simulink model "bingo_dec16_32k"  (R2018a)
settings: Solver=VariableStepDiscrete  StartTime=0.0  StopTime=10.0  RelTol=1e-3
undefined symbols (not defined in the file): pfb_coeff_gen_calc
libraries: xbsIndex_r4 x9772, casper_library_misc x15, xps_library x4, casper_library_delays x2
(part 3 of 49)

== system bingo_dec16_32k/bit_sel_xy_re ==
  shift : Inport
  sync : Inport  Port=2
  din64 : Inport  Port=3
  valid : Inport  Port=4
  Reinterpret : xbsIndex_r4/Reinterpret  force_arith_type=on  arith_type=Unsigned  force_bin_pt=on  bin_pt=0  block_type=reinterpret
  Terminator{1..32} (32 alike) : Terminator
  barrel_switcher : Subsystem  AncestorBlock=casper_library_reorder/barrel_switcher  mask(barrel_switcher){n_inputs=6, async=off}
      mask prompts: n_inputs "Number of Inputs: (2^?)"; async "Asynchronous operation"
      mask help:
      | Shifts input to right by amount specified on sel,
      | wrapping around into higher order bits.
      mask init:
      | barrel_switcher_init(gcb,...
      |     'n_inputs', n_inputs, ...
      |     'async', async);
      mask Help: eval('xlWeb(''http://casper.berkeley.edu/wiki/Barrel_switcher'')')
  bus_create : Subsystem  AncestorBlock=casper_library_flow_control/bus_create  mask(bus_create){inputNum=32}
      mask prompts: inputNum "Number of inputs:"
      mask init:
      | bus_create_init(gcb,...
      |     'inputNum', inputNum);
  bus_expand1 : Subsystem  AncestorBlock=casper_library_flow_control/bus_expand  mask(bus_expand){mode=divisions of equal size, outputNum=64, outputWidth=1, outputBinaryPt=0, outputArithmeticType=0, show_format=off, outputToWorkspace=off, variablePrefix=out, outputToModelAsWell=on}
      mask prompts: outputNum "Number of outputs:"; outputWidth "Output width:"; outputBinaryPt "Output binary point position:"; outputArithmeticType "Output arithmetic type (ufix=0, fix=1, bool=2):"; show_format "Print format string?"; outputToWorkspace "Output to workspace?"; variablePrefix "Variable name prefix:"; outputToModelAsWell "Output to model as well?"
      mask help:
      | Expands a 'bus' made using a bus_create or Xilinx
      | concat block.
      | The input will be divided into the specified number
      | of outputs with the specified arithmetic types.
      | Divisions are made from most significant bit.
      mask init: same as bingo_dec16_32k/bit_sel_xx/bus_expand1
      settings: AttributesFormatString=64 outputs
      mask TypeOptions mode: divisions of equal size | divisions of arbitrary size
      mask Callback mode: bus_expand_callback();
      mask Callback outputWidth: bus_expand_callback();
      mask Callback outputToWorkspace: bus_expand_callback();
  sync_out : Outport
  "dout32 " : Outport  Port=2
  valid_out : Outport  Port=3
  wires:
  bus_expand1/13(out52) -> barrel_switcher/15(In13)
  bus_expand1/42(out23) -> barrel_switcher/44(In42)
  bus_expand1/27(out38) -> barrel_switcher/29(In27)
  bus_expand1/26(out39) -> barrel_switcher/28(In26)
  bus_expand1/33(out32) -> barrel_switcher/35(In33)
  bus_expand1/44(out21) -> barrel_switcher/46(In44)
  bus_expand1/12(out53) -> barrel_switcher/14(In12)
  bus_expand1/35(out30) -> barrel_switcher/37(In35)
  bus_expand1/23(out42) -> barrel_switcher/25(In23)
  bus_expand1/45(out20) -> barrel_switcher/47(In45)
  bus_expand1/50(out15) -> barrel_switcher/52(In50)
  bus_expand1/56(out9) -> barrel_switcher/58(In56)
  sync/1 -> barrel_switcher/2(sync_in)
  bus_expand1/24(out41) -> barrel_switcher/26(In24)
  bus_expand1/58(out7) -> barrel_switcher/60(In58)
  bus_expand1/53(out12) -> barrel_switcher/55(In53)
  bus_expand1/29(out36) -> barrel_switcher/31(In29)
  bus_expand1/43(out22) -> barrel_switcher/45(In43)
  bus_expand1/3(out62) -> barrel_switcher/5(In3)
  bus_expand1/61(out4) -> barrel_switcher/63(In61)
  bus_expand1/1(msb_out64) -> barrel_switcher/3(In1)
  bus_expand1/28(out37) -> barrel_switcher/30(In28)
  Reinterpret/1 -> bus_expand1/1(bus_in)
  bus_expand1/8(out57) -> barrel_switcher/10(In8)
  bus_expand1/20(out45) -> barrel_switcher/22(In20)
  bus_expand1/59(out6) -> barrel_switcher/61(In59)
  bus_expand1/30(out35) -> barrel_switcher/32(In30)
  bus_expand1/19(out46) -> barrel_switcher/21(In19)
  bus_expand1/9(out56) -> barrel_switcher/11(In9)
  bus_expand1/11(out54) -> barrel_switcher/13(In11)
  bus_expand1/18(out47) -> barrel_switcher/20(In18)
  bus_expand1/25(out40) -> barrel_switcher/27(In25)
  bus_expand1/32(out33) -> barrel_switcher/34(In32)
  bus_expand1/62(out3) -> barrel_switcher/64(In62)
  bus_expand1/37(out28) -> barrel_switcher/39(In37)
  bus_expand1/36(out29) -> barrel_switcher/38(In36)
  bus_expand1/41(out24) -> barrel_switcher/43(In41)
  bus_expand1/22(out43) -> barrel_switcher/24(In22)
  bus_expand1/48(out17) -> barrel_switcher/50(In48)
  bus_expand1/7(out58) -> barrel_switcher/9(In7)
  bus_expand1/63(out2) -> barrel_switcher/65(In63)
  bus_expand1/15(out50) -> barrel_switcher/17(In15)
  bus_expand1/49(out16) -> barrel_switcher/51(In49)
  shift/1 -> barrel_switcher/1(sel)
  bus_expand1/21(out44) -> barrel_switcher/23(In21)
  bus_expand1/46(out19) -> barrel_switcher/48(In46)
  bus_expand1/52(out13) -> barrel_switcher/54(In52)
  bus_expand1/54(out11) -> barrel_switcher/56(In54)
  bus_expand1/4(out61) -> barrel_switcher/6(In4)
  bus_expand1/31(out34) -> barrel_switcher/33(In31)
  bus_expand1/40(out25) -> barrel_switcher/42(In40)
  bus_expand1/39(out26) -> barrel_switcher/41(In39)
  bus_expand1/51(out14) -> barrel_switcher/53(In51)
  bus_expand1/64(lsb_out1) -> barrel_switcher/66(In64)
  bus_expand1/38(out27) -> barrel_switcher/40(In38)
  din64/1 -> Reinterpret/1
  bus_expand1/5(out60) -> barrel_switcher/7(In5)
  bus_expand1/17(out48) -> barrel_switcher/19(In17)
  bus_expand1/16(out49) -> barrel_switcher/18(In16)
  bus_expand1/10(out55) -> barrel_switcher/12(In10)
  bus_expand1/14(out51) -> barrel_switcher/16(In14)
  bus_expand1/2(out63) -> barrel_switcher/4(In2)
  bus_expand1/60(out5) -> barrel_switcher/62(In60)
  bus_expand1/55(out10) -> barrel_switcher/57(In55)
  bus_expand1/6(out59) -> barrel_switcher/8(In6)
  bus_expand1/47(out18) -> barrel_switcher/49(In47)
  bus_expand1/57(out8) -> barrel_switcher/59(In57)
  bus_expand1/34(out31) -> barrel_switcher/36(In34)
  bus_create/1(bus_out) -> "dout32 "/1
  barrel_switcher/1(sync_out) -> sync_out/1
  barrel_switcher/66(valid_out) -> valid_out/1
  valid/1 -> barrel_switcher/67(valid_in)
  barrel_switcher/35(Out34) -> Terminator1/1
  barrel_switcher/40(Out39) -> Terminator7/1
  barrel_switcher/45(Out44) -> Terminator11/1
  barrel_switcher/56(Out55) -> Terminator30/1
  barrel_switcher/42(Out41) -> Terminator9/1
  barrel_switcher/64(Out63) -> Terminator24/1
  barrel_switcher/47(Out46) -> Terminator13/1
  barrel_switcher/58(Out57) -> Terminator32/1
  barrel_switcher/61(Out60) -> Terminator19/1
  barrel_switcher/37(Out36) -> Terminator2/1
  barrel_switcher/36(Out35) -> Terminator3/1
  barrel_switcher/53(Out52) -> Terminator25/1
  barrel_switcher/51(Out50) -> Terminator17/1
  barrel_switcher/43(Out42) -> Terminator8/1
  barrel_switcher/62(Out61) -> Terminator22/1
  barrel_switcher/50(Out49) -> Terminator18/1
  barrel_switcher/57(Out56) -> Terminator29/1
  barrel_switcher/49(Out48) -> Terminator15/1
  barrel_switcher/55(Out54) -> Terminator27/1
  barrel_switcher/52(Out51) -> Terminator26/1
  barrel_switcher/60(Out59) -> Terminator20/1
  barrel_switcher/46(Out45) -> Terminator14/1
  barrel_switcher/63(Out62) -> Terminator21/1
  barrel_switcher/65(Out64) -> Terminator23/1
  barrel_switcher/34(Out33) -> Terminator10/1
  barrel_switcher/54(Out53) -> Terminator28/1
  barrel_switcher/41(Out40) -> Terminator6/1
  barrel_switcher/59(Out58) -> Terminator31/1
  barrel_switcher/38(Out37) -> Terminator5/1
  barrel_switcher/44(Out43) -> Terminator12/1
  barrel_switcher/39(Out38) -> Terminator4/1
  barrel_switcher/48(Out47) -> Terminator16/1
  barrel_switcher/2(Out1) -> bus_create/1(in1)
  barrel_switcher/3(Out2) -> bus_create/2(in2)
  barrel_switcher/4(Out3) -> bus_create/3(in3)
  barrel_switcher/5(Out4) -> bus_create/4(in4)
  barrel_switcher/6(Out5) -> bus_create/5(in5)
  barrel_switcher/7(Out6) -> bus_create/6(in6)
  barrel_switcher/8(Out7) -> bus_create/7(in7)
  barrel_switcher/9(Out8) -> bus_create/8(in8)
  barrel_switcher/10(Out9) -> bus_create/9(in9)
  barrel_switcher/11(Out10) -> bus_create/10(in10)
  barrel_switcher/12(Out11) -> bus_create/11(in11)
  barrel_switcher/13(Out12) -> bus_create/12(in12)
  barrel_switcher/14(Out13) -> bus_create/13(in13)
  barrel_switcher/15(Out14) -> bus_create/14(in14)
  barrel_switcher/16(Out15) -> bus_create/15(in15)
  barrel_switcher/17(Out16) -> bus_create/16(in16)
  barrel_switcher/18(Out17) -> bus_create/17(in17)
  barrel_switcher/19(Out18) -> bus_create/18(in18)
  barrel_switcher/20(Out19) -> bus_create/19(in19)
  barrel_switcher/21(Out20) -> bus_create/20(in20)
  barrel_switcher/22(Out21) -> bus_create/21(in21)
  barrel_switcher/23(Out22) -> bus_create/22(in22)
  barrel_switcher/24(Out23) -> bus_create/23(in23)
  barrel_switcher/25(Out24) -> bus_create/24(in24)
  barrel_switcher/26(Out25) -> bus_create/25(in25)
  barrel_switcher/27(Out26) -> bus_create/26(in26)
  barrel_switcher/28(Out27) -> bus_create/27(in27)
  barrel_switcher/29(Out28) -> bus_create/28(in28)
  barrel_switcher/30(Out29) -> bus_create/29(in29)
  barrel_switcher/31(Out30) -> bus_create/30(in30)
  barrel_switcher/32(Out31) -> bus_create/31(in31)
  barrel_switcher/33(Out32) -> bus_create/32(in32)

== system bingo_dec16_32k/bit_sel_yy ==
  shift : Inport
  sync : Inport  Port=2
  din64 : Inport  Port=3
  valid : Inport  Port=4
  Reinterpret : xbsIndex_r4/Reinterpret  force_arith_type=on  arith_type=Unsigned  force_bin_pt=on  bin_pt=0  block_type=reinterpret
  Terminator{1..32} (32 alike) : Terminator
  barrel_switcher : Subsystem  AncestorBlock=casper_library_reorder/barrel_switcher  mask(barrel_switcher){n_inputs=6, async=off}
      mask prompts: n_inputs "Number of Inputs: (2^?)"; async "Asynchronous operation"
      mask help:
      | Shifts input to right by amount specified on sel,
      | wrapping around into higher order bits.
      mask init:
      | barrel_switcher_init(gcb,...
      |     'n_inputs', n_inputs, ...
      |     'async', async);
      mask Help: eval('xlWeb(''http://casper.berkeley.edu/wiki/Barrel_switcher'')')
  bus_create : Subsystem  AncestorBlock=casper_library_flow_control/bus_create  mask(bus_create){inputNum=32}
      mask prompts: inputNum "Number of inputs:"
      mask init:
      | bus_create_init(gcb,...
      |     'inputNum', inputNum);
  bus_expand1 : Subsystem  AncestorBlock=casper_library_flow_control/bus_expand  mask(bus_expand){mode=divisions of equal size, outputNum=64, outputWidth=1, outputBinaryPt=0, outputArithmeticType=0, show_format=off, outputToWorkspace=off, variablePrefix=out, outputToModelAsWell=on}
      mask prompts: outputNum "Number of outputs:"; outputWidth "Output width:"; outputBinaryPt "Output binary point position:"; outputArithmeticType "Output arithmetic type (ufix=0, fix=1, bool=2):"; show_format "Print format string?"; outputToWorkspace "Output to workspace?"; variablePrefix "Variable name prefix:"; outputToModelAsWell "Output to model as well?"
      mask help:
      | Expands a 'bus' made using a bus_create or Xilinx
      | concat block.
      | The input will be divided into the specified number
      | of outputs with the specified arithmetic types.
      | Divisions are made from most significant bit.
      mask init: same as bingo_dec16_32k/bit_sel_xx/bus_expand1
      settings: AttributesFormatString=64 outputs
      mask TypeOptions mode: divisions of equal size | divisions of arbitrary size
      mask Callback mode: bus_expand_callback();
      mask Callback outputWidth: bus_expand_callback();
      mask Callback outputToWorkspace: bus_expand_callback();
  sync_out : Outport
  "dout32 " : Outport  Port=2
  valid_out : Outport  Port=3
  wires:
  bus_expand1/13(out52) -> barrel_switcher/15(In13)
  bus_expand1/42(out23) -> barrel_switcher/44(In42)
  bus_expand1/27(out38) -> barrel_switcher/29(In27)
  bus_expand1/26(out39) -> barrel_switcher/28(In26)
  bus_expand1/33(out32) -> barrel_switcher/35(In33)
  bus_expand1/44(out21) -> barrel_switcher/46(In44)
  bus_expand1/12(out53) -> barrel_switcher/14(In12)
  bus_expand1/35(out30) -> barrel_switcher/37(In35)
  bus_expand1/23(out42) -> barrel_switcher/25(In23)
  bus_expand1/45(out20) -> barrel_switcher/47(In45)
  bus_expand1/50(out15) -> barrel_switcher/52(In50)
  bus_expand1/56(out9) -> barrel_switcher/58(In56)
  sync/1 -> barrel_switcher/2(sync_in)
  bus_expand1/24(out41) -> barrel_switcher/26(In24)
  bus_expand1/58(out7) -> barrel_switcher/60(In58)
  bus_expand1/53(out12) -> barrel_switcher/55(In53)
  bus_expand1/29(out36) -> barrel_switcher/31(In29)
  bus_expand1/43(out22) -> barrel_switcher/45(In43)
  bus_expand1/3(out62) -> barrel_switcher/5(In3)
  bus_expand1/61(out4) -> barrel_switcher/63(In61)
  bus_expand1/1(msb_out64) -> barrel_switcher/3(In1)
  bus_expand1/28(out37) -> barrel_switcher/30(In28)
  Reinterpret/1 -> bus_expand1/1(bus_in)
  bus_expand1/8(out57) -> barrel_switcher/10(In8)
  bus_expand1/20(out45) -> barrel_switcher/22(In20)
  bus_expand1/59(out6) -> barrel_switcher/61(In59)
  bus_expand1/30(out35) -> barrel_switcher/32(In30)
  bus_expand1/19(out46) -> barrel_switcher/21(In19)
  bus_expand1/9(out56) -> barrel_switcher/11(In9)
  bus_expand1/11(out54) -> barrel_switcher/13(In11)
  bus_expand1/18(out47) -> barrel_switcher/20(In18)
  bus_expand1/25(out40) -> barrel_switcher/27(In25)
  bus_expand1/32(out33) -> barrel_switcher/34(In32)
  bus_expand1/62(out3) -> barrel_switcher/64(In62)
  bus_expand1/37(out28) -> barrel_switcher/39(In37)
  bus_expand1/36(out29) -> barrel_switcher/38(In36)
  bus_expand1/41(out24) -> barrel_switcher/43(In41)
  bus_expand1/22(out43) -> barrel_switcher/24(In22)
  bus_expand1/48(out17) -> barrel_switcher/50(In48)
  bus_expand1/7(out58) -> barrel_switcher/9(In7)
  bus_expand1/63(out2) -> barrel_switcher/65(In63)
  bus_expand1/15(out50) -> barrel_switcher/17(In15)
  bus_expand1/49(out16) -> barrel_switcher/51(In49)
  shift/1 -> barrel_switcher/1(sel)
  bus_expand1/21(out44) -> barrel_switcher/23(In21)
  bus_expand1/46(out19) -> barrel_switcher/48(In46)
  bus_expand1/52(out13) -> barrel_switcher/54(In52)
  bus_expand1/54(out11) -> barrel_switcher/56(In54)
  bus_expand1/4(out61) -> barrel_switcher/6(In4)
  bus_expand1/31(out34) -> barrel_switcher/33(In31)
  bus_expand1/40(out25) -> barrel_switcher/42(In40)
  bus_expand1/39(out26) -> barrel_switcher/41(In39)
  bus_expand1/51(out14) -> barrel_switcher/53(In51)
  bus_expand1/64(lsb_out1) -> barrel_switcher/66(In64)
  bus_expand1/38(out27) -> barrel_switcher/40(In38)
  din64/1 -> Reinterpret/1
  bus_expand1/5(out60) -> barrel_switcher/7(In5)
  bus_expand1/17(out48) -> barrel_switcher/19(In17)
  bus_expand1/16(out49) -> barrel_switcher/18(In16)
  bus_expand1/10(out55) -> barrel_switcher/12(In10)
  bus_expand1/14(out51) -> barrel_switcher/16(In14)
  bus_expand1/2(out63) -> barrel_switcher/4(In2)
  bus_expand1/60(out5) -> barrel_switcher/62(In60)
  bus_expand1/55(out10) -> barrel_switcher/57(In55)
  bus_expand1/6(out59) -> barrel_switcher/8(In6)
  bus_expand1/47(out18) -> barrel_switcher/49(In47)
  bus_expand1/57(out8) -> barrel_switcher/59(In57)
  bus_expand1/34(out31) -> barrel_switcher/36(In34)
  bus_create/1(bus_out) -> "dout32 "/1
  barrel_switcher/1(sync_out) -> sync_out/1
  barrel_switcher/66(valid_out) -> valid_out/1
  valid/1 -> barrel_switcher/67(valid_in)
  barrel_switcher/35(Out34) -> Terminator1/1
  barrel_switcher/40(Out39) -> Terminator7/1
  barrel_switcher/45(Out44) -> Terminator11/1
  barrel_switcher/56(Out55) -> Terminator30/1
  barrel_switcher/42(Out41) -> Terminator9/1
  barrel_switcher/64(Out63) -> Terminator24/1
  barrel_switcher/47(Out46) -> Terminator13/1
  barrel_switcher/58(Out57) -> Terminator32/1
  barrel_switcher/61(Out60) -> Terminator19/1
  barrel_switcher/37(Out36) -> Terminator2/1
  barrel_switcher/36(Out35) -> Terminator3/1
  barrel_switcher/53(Out52) -> Terminator25/1
  barrel_switcher/51(Out50) -> Terminator17/1
  barrel_switcher/43(Out42) -> Terminator8/1
  barrel_switcher/62(Out61) -> Terminator22/1
  barrel_switcher/50(Out49) -> Terminator18/1
  barrel_switcher/57(Out56) -> Terminator29/1
  barrel_switcher/49(Out48) -> Terminator15/1
  barrel_switcher/55(Out54) -> Terminator27/1
  barrel_switcher/52(Out51) -> Terminator26/1
  barrel_switcher/60(Out59) -> Terminator20/1
  barrel_switcher/46(Out45) -> Terminator14/1
  barrel_switcher/63(Out62) -> Terminator21/1
  barrel_switcher/65(Out64) -> Terminator23/1
  barrel_switcher/34(Out33) -> Terminator10/1
  barrel_switcher/54(Out53) -> Terminator28/1
  barrel_switcher/41(Out40) -> Terminator6/1
  barrel_switcher/59(Out58) -> Terminator31/1
  barrel_switcher/38(Out37) -> Terminator5/1
  barrel_switcher/44(Out43) -> Terminator12/1
  barrel_switcher/39(Out38) -> Terminator4/1
  barrel_switcher/48(Out47) -> Terminator16/1
  barrel_switcher/2(Out1) -> bus_create/1(in1)
  barrel_switcher/3(Out2) -> bus_create/2(in2)
  barrel_switcher/4(Out3) -> bus_create/3(in3)
  barrel_switcher/5(Out4) -> bus_create/4(in4)
  barrel_switcher/6(Out5) -> bus_create/5(in5)
  barrel_switcher/7(Out6) -> bus_create/6(in6)
  barrel_switcher/8(Out7) -> bus_create/7(in7)
  barrel_switcher/9(Out8) -> bus_create/8(in8)
  barrel_switcher/10(Out9) -> bus_create/9(in9)
  barrel_switcher/11(Out10) -> bus_create/10(in10)
  barrel_switcher/12(Out11) -> bus_create/11(in11)
  barrel_switcher/13(Out12) -> bus_create/12(in12)
  barrel_switcher/14(Out13) -> bus_create/13(in13)
  barrel_switcher/15(Out14) -> bus_create/14(in14)
  barrel_switcher/16(Out15) -> bus_create/15(in15)
  barrel_switcher/17(Out16) -> bus_create/16(in16)
  barrel_switcher/18(Out17) -> bus_create/17(in17)
  barrel_switcher/19(Out18) -> bus_create/18(in18)
  barrel_switcher/20(Out19) -> bus_create/19(in19)
  barrel_switcher/21(Out20) -> bus_create/20(in20)
  barrel_switcher/22(Out21) -> bus_create/21(in21)
  barrel_switcher/23(Out22) -> bus_create/22(in22)
  barrel_switcher/24(Out23) -> bus_create/23(in23)
  barrel_switcher/25(Out24) -> bus_create/24(in24)
  barrel_switcher/26(Out25) -> bus_create/25(in25)
  barrel_switcher/27(Out26) -> bus_create/26(in26)
  barrel_switcher/28(Out27) -> bus_create/27(in27)
  barrel_switcher/29(Out28) -> bus_create/28(in28)
  barrel_switcher/30(Out29) -> bus_create/29(in29)
  barrel_switcher/31(Out30) -> bus_create/30(in30)
  barrel_switcher/32(Out31) -> bus_create/31(in31)
  barrel_switcher/33(Out32) -> bus_create/32(in32)

== system bingo_dec16_32k/bus_create ==
  in1 : Inport
  in2 : Inport  Port=2
  in3 : Inport  Port=3
  in4 : Inport  Port=4
  concatenate : xbsIndex_r4/Concat  num_inputs=4  dbl_ovrd=off  block_type=concat
  reinterpret{1..4} (4 alike) : xbsIndex_r4/Reinterpret  force_arith_type=on  arith_type=Unsigned  force_bin_pt=on  bin_pt=0  block_type=reinterpret
      reinterpret1 settings: infoedit="Changes signal type without altering the binary representation.   You can changed the signal between signed and unsigned, and relocate the binary point.<br><br>Hardware notes: In hardware this block costs nothing.<br><br>Example:  Suppose the input is 6 bits wide, signed, with 2 fractional bits, and the output is forced to unsigned with 0 fractional bits.  Then an input of -2.0 (1110.00 in binary 2's complement) becomes an output of 56 (111000 in binary)."
      reinterpret2 settings: infoedit="Changes signal type without altering the binary representation.   You can changed the signal between signed and unsigned, and relocate the binary point.<br><br>Hardware notes: In hardware this block costs nothing.<br><br>Example:  Suppose the input is 6 bits wide, signed, with 2 fractional bits, and the output is forced to unsigned with 0 fractional bits.  Then an input of -2.0 (1110.00 in binary 2's complement) becomes an output of 56 (111000 in binary)."
  bus_out : Outport
  wires:
  concatenate/1 -> bus_out/1
  in1/1 -> reinterpret1/1
  reinterpret1/1 -> concatenate/1
  in2/1 -> reinterpret2/1
  reinterpret2/1 -> concatenate/2
  in3/1 -> reinterpret3/1
  reinterpret3/1 -> concatenate/3
  in4/1 -> reinterpret4/1
  reinterpret4/1 -> concatenate/4

== system bingo_dec16_32k/calc_adc_sum_sq1 ==
  In1 : Inport
  In2 : Inport  Port=2
  "valid " : Inport  Port=3
  Accumulator : xbsIndex_r4/Accumulator  operation=Add  n_bits=47  overflow=Wrap  scale=1  rst=on  hasbypass=on  infoeditControl=reset for floating point data type must be asserted for a minimum of 2 cycles  en=on  latency=0  msb_inp=100  msb=100  lsb=-100  use_behavioral_HDL=off  implementation=DSP48  dbl_ovrd=off  block_type=accum
      settings: xl_area=[0, 0, 0, 0, 0, 0, 0]  block_version=10.1.3
  AddSub9 : xbsIndex_r4/AddSub  mode=Addition  use_carryin=off  use_carryout=off  en=off  latency=1  precision=Full  arith_type=Unsigned  n_bits=16  bin_pt=14  quantization=Truncate  overflow=Wrap  use_behavioral_HDL=off  hw_selection=Fabric  pipelined=off  dbl_ovrd=off  block_type=addsub
  Convert1 : xbsIndex_r4/Convert  gui_display_data_type=Fixed-point  arith_type=Unsigned  n_bits=32  bin_pt=15  float_type=Single  exp_bits=8  fraction_bits=24  quantization=Truncate  overflow=Wrap  en=off  latency=0  pipeline=off  dbl_ovrd=off  block_type=convert
      settings: block_version=11.4
  Counter1 : xbsIndex_r4/Counter  cnt_type=Free Running  cnt_to=Inf  operation=Up  start_count=0  cnt_by_val=1  arith_type=Unsigned  n_bits=16  bin_pt=0  load_pin=off  rst=off  en=on  explicit_period=on  period=1  use_behavioral_HDL=off  implementation=DSP48  use_rpm=on  dbl_ovrd=off  block_type=counter
      settings: xl_area=[0, 0, 0, 0, 0, 0, 0]
  Delay : xbsIndex_r4/Delay  rst=off  infoeditControl=Selection of Reset will increase slice count due to use of real FFs and instead of SRLs  en=off  latency=3  reg_retiming=off  dbl_ovrd=off  block_type=delay
  Delay1 : xbsIndex_r4/Delay  rst=off  infoeditControl=Selection of Reset will increase slice count due to use of real FFs and instead of SRLs  en=off  latency=2  reg_retiming=on  dbl_ovrd=off  block_type=delay
      settings: block_version=11.4
  Logical : xbsIndex_r4/Logical  logical_function=AND  inputs=2  en=off  latency=0  precision=Full  arith_type=Unsigned  n_bits=16  bin_pt=0  align_bp=on  dbl_ovrd=off  block_type=logical
  Mult : xbsIndex_r4/Mult  precision=Full  arith_type="Signed  (2's comp)"  n_bits=8  bin_pt=2  quantization=Truncate  overflow=Wrap  en=off  latency=2  use_behavioral_HDL=on  opt=Speed  use_embedded=on  optimum_pipeline=off  pipeline=on  dbl_ovrd=off  use_rpm=on  placement_style=Rectangular shape  block_type=mult
      settings: xl_area=[0, 0, 0, 0, 0, 0, 0]  block_version=10.1.3
  Mult8 : xbsIndex_r4/Mult  precision=Full  arith_type="Signed  (2's comp)"  n_bits=8  bin_pt=2  quantization=Truncate  overflow=Wrap  en=off  latency=2  use_behavioral_HDL=on  opt=Speed  use_embedded=on  optimum_pipeline=off  pipeline=on  dbl_ovrd=off  use_rpm=on  placement_style=Rectangular shape  block_type=mult
      settings: xl_area=[0, 0, 0, 0, 0, 0, 0]  block_version=10.1.3
  Register : xbsIndex_r4/Register  init=0  rst=off  en=on  dbl_ovrd=off  block_type=register
      settings: xl_area=[0, 0, 0, 0, 0, 0, 0]
  Slice : xbsIndex_r4/Slice  nbits=1  boolean_output=off  mode=Upper Bit Location + Width  bit1=0  base1=MSB of Input  bit0=0  base0=LSB of Input  dbl_ovrd=off  block_type=slice
      settings: infoedit="Extracts a given range of bits from each input sample and presents it at the output.  The output type is ordinarily unsigned with binary point at zero, but can be Boolean when the slice is one bit wide.<P><P>Hardware notes: In hardware this block costs nothing."  block_version=10.1.3
  negedge : Subsystem
  sum_sq : Outport
  wires:
  Accumulator/1 -> Register/1
  Register/1 -> Convert1/1
  In2/1 -> Mult/1, Mult/2
  Counter1/1 -> Slice/1
  Slice/1 -> negedge/1(In)
  negedge/1(Out1) -> Delay1/1
  Convert1/1 -> sum_sq/1
  AddSub9/1 -> Accumulator/1
  Delay1/1 -> Logical/2
  In1/1 -> Mult8/1, Mult8/2
  Mult8/1 -> AddSub9/1
  Mult/1 -> AddSub9/2
  "valid "/1 -> Counter1/1, Delay/1
  Delay/1 -> Logical/1, Accumulator/3
  Logical/1 -> Register/2, Accumulator/2

== system bingo_dec16_32k/calc_adc_sum_sq2 ==
  In1 : Inport
  In2 : Inport  Port=2
  "valid " : Inport  Port=3
  Accumulator : xbsIndex_r4/Accumulator  operation=Add  n_bits=47  overflow=Wrap  scale=1  rst=on  hasbypass=on  infoeditControl=reset for floating point data type must be asserted for a minimum of 2 cycles  en=on  latency=0  msb_inp=100  msb=100  lsb=-100  use_behavioral_HDL=off  implementation=DSP48  dbl_ovrd=off  block_type=accum
      settings: xl_area=[0, 0, 0, 0, 0, 0, 0]  block_version=10.1.3
  AddSub9 : xbsIndex_r4/AddSub  mode=Addition  use_carryin=off  use_carryout=off  en=off  latency=1  precision=Full  arith_type=Unsigned  n_bits=16  bin_pt=14  quantization=Truncate  overflow=Wrap  use_behavioral_HDL=off  hw_selection=Fabric  pipelined=off  dbl_ovrd=off  block_type=addsub
  Convert1 : xbsIndex_r4/Convert  gui_display_data_type=Fixed-point  arith_type=Unsigned  n_bits=32  bin_pt=15  float_type=Single  exp_bits=8  fraction_bits=24  quantization=Truncate  overflow=Wrap  en=off  latency=0  pipeline=off  dbl_ovrd=off  block_type=convert
      settings: block_version=11.4
  Counter1 : xbsIndex_r4/Counter  cnt_type=Free Running  cnt_to=Inf  operation=Up  start_count=0  cnt_by_val=1  arith_type=Unsigned  n_bits=16  bin_pt=0  load_pin=off  rst=off  en=on  explicit_period=on  period=1  use_behavioral_HDL=off  implementation=DSP48  use_rpm=on  dbl_ovrd=off  block_type=counter
      settings: xl_area=[0, 0, 0, 0, 0, 0, 0]
  Delay : xbsIndex_r4/Delay  rst=off  infoeditControl=Selection of Reset will increase slice count due to use of real FFs and instead of SRLs  en=off  latency=3  reg_retiming=off  dbl_ovrd=off  block_type=delay
  Delay1 : xbsIndex_r4/Delay  rst=off  infoeditControl=Selection of Reset will increase slice count due to use of real FFs and instead of SRLs  en=off  latency=2  reg_retiming=on  dbl_ovrd=off  block_type=delay
      settings: block_version=11.4
  Logical : xbsIndex_r4/Logical  logical_function=AND  inputs=2  en=off  latency=0  precision=Full  arith_type=Unsigned  n_bits=16  bin_pt=0  align_bp=on  dbl_ovrd=off  block_type=logical
  Mult : xbsIndex_r4/Mult  precision=Full  arith_type="Signed  (2's comp)"  n_bits=8  bin_pt=2  quantization=Truncate  overflow=Wrap  en=off  latency=2  use_behavioral_HDL=on  opt=Speed  use_embedded=on  optimum_pipeline=off  pipeline=on  dbl_ovrd=off  use_rpm=on  placement_style=Rectangular shape  block_type=mult
      settings: xl_area=[0, 0, 0, 0, 0, 0, 0]  block_version=10.1.3
  Mult8 : xbsIndex_r4/Mult  precision=Full  arith_type="Signed  (2's comp)"  n_bits=8  bin_pt=2  quantization=Truncate  overflow=Wrap  en=off  latency=2  use_behavioral_HDL=on  opt=Speed  use_embedded=on  optimum_pipeline=off  pipeline=on  dbl_ovrd=off  use_rpm=on  placement_style=Rectangular shape  block_type=mult
      settings: xl_area=[0, 0, 0, 0, 0, 0, 0]  block_version=10.1.3
  Register : xbsIndex_r4/Register  init=0  rst=off  en=on  dbl_ovrd=off  block_type=register
      settings: xl_area=[0, 0, 0, 0, 0, 0, 0]
  Slice : xbsIndex_r4/Slice  nbits=1  boolean_output=off  mode=Upper Bit Location + Width  bit1=0  base1=MSB of Input  bit0=0  base0=LSB of Input  dbl_ovrd=off  block_type=slice
      settings: infoedit="Extracts a given range of bits from each input sample and presents it at the output.  The output type is ordinarily unsigned with binary point at zero, but can be Boolean when the slice is one bit wide.<P><P>Hardware notes: In hardware this block costs nothing."  block_version=10.1.3
  negedge : Subsystem
  sum_sq : Outport
  wires:
  Accumulator/1 -> Register/1
  Register/1 -> Convert1/1
  In2/1 -> Mult/1, Mult/2
  Counter1/1 -> Slice/1
  Slice/1 -> negedge/1(In)
  negedge/1(Out1) -> Delay1/1
  Convert1/1 -> sum_sq/1
  AddSub9/1 -> Accumulator/1
  Delay1/1 -> Logical/2
  In1/1 -> Mult8/1, Mult8/2
  Mult8/1 -> AddSub9/1
  Mult/1 -> AddSub9/2
  "valid "/1 -> Counter1/1, Delay/1
  Delay/1 -> Logical/1, Accumulator/3
  Logical/1 -> Register/2, Accumulator/2

== system bingo_dec16_32k/center_freq ==
  sim_1 : Inport
  bingo_dec16_32k_center_freq_user_data_out : xbsIndex_r4/Gateway In  gui_display_data_type=Fixed-point  arith_type=Unsigned  n_bits=32  bin_pt=0  preci_type=Single  exp_width=8  frac_width=24  rows=1  columns=1  quantization="Round  (unbiased: +/- Inf)"  overflow=Saturate  period=1  UseAsADC=off  ADCChannel='1'  interface=None  automatic_assignment=on  address_offset=hex2dec('00')  intf_name=''  intf_description=''  default_value=0  timing_constraint=None  locs_specified=off  LOCs={}  io_standard={}  inherit_from_input=off  hdl_port=on  dbl_ovrd=off  block_type=gatewayin
  convert1_1 : DataTypeConversion  OutDataTypeStr=fixdt('ufix32_En0')  LockScale=on
  convert2_1 : DataTypeConversion  OutDataTypeStr=fixdt('ufix32_En0')  ConvertRealWorld=Stored Integer (SI)  LockScale=on
  gain_1 : Gain
  io_delay : xbsIndex_r4/Delay  rst=off  infoeditControl=Selection of Reset will increase slice count due to use of real FFs and instead of SRLs  en=off  latency=0  reg_retiming=on  dbl_ovrd=off  block_type=delay
  reint1 : xbsIndex_r4/Reinterpret  force_arith_type=on  arith_type=Unsigned  force_bin_pt=on  bin_pt=0  block_type=reinterpret
  slice_reg : xbsIndex_r4/Slice  nbits=32  boolean_output=off  mode=Lower Bit Location + Width  bit1=0  base1=MSB of Input  bit0=0  base0=LSB of Input  dbl_ovrd=off  block_type=slice
  in_reg : Outport
  wires:
  bingo_dec16_32k_center_freq_user_data_out/1 -> io_delay/1
  sim_1/1 -> convert1_1/1
  convert1_1/1 -> convert2_1/1
  convert2_1/1 -> gain_1/1
  gain_1/1 -> bingo_dec16_32k_center_freq_user_data_out/1
  io_delay/1 -> slice_reg/1
  slice_reg/1 -> reint1/1
  reint1/1 -> in_reg/1

== system bingo_dec16_32k/clr_bc ==
  sim_1 : Inport
  bingo_dec16_32k_clr_bc_user_data_out : xbsIndex_r4/Gateway In  gui_display_data_type=Fixed-point  arith_type=Unsigned  n_bits=32  bin_pt=0  preci_type=Single  exp_width=8  frac_width=24  rows=1  columns=1  quantization="Round  (unbiased: +/- Inf)"  overflow=Saturate  period=1  UseAsADC=off  ADCChannel='1'  interface=None  automatic_assignment=on  address_offset=hex2dec('00')  intf_name=''  intf_description=''  default_value=0  timing_constraint=None  locs_specified=off  LOCs={}  io_standard={}  inherit_from_input=off  hdl_port=on  dbl_ovrd=off  block_type=gatewayin
  convert1_1 : DataTypeConversion  OutDataTypeStr=fixdt('ufix32_En0')  LockScale=on
  convert2_1 : DataTypeConversion  OutDataTypeStr=fixdt('ufix32_En0')  ConvertRealWorld=Stored Integer (SI)  LockScale=on
  gain_1 : Gain
  io_delay : xbsIndex_r4/Delay  rst=off  infoeditControl=Selection of Reset will increase slice count due to use of real FFs and instead of SRLs  en=off  latency=0  reg_retiming=on  dbl_ovrd=off  block_type=delay
  reint1 : xbsIndex_r4/Reinterpret  force_arith_type=on  arith_type=Unsigned  force_bin_pt=on  bin_pt=0  block_type=reinterpret
  slice_reg : xbsIndex_r4/Slice  nbits=32  boolean_output=off  mode=Lower Bit Location + Width  bit1=0  base1=MSB of Input  bit0=0  base0=LSB of Input  dbl_ovrd=off  block_type=slice
  in_reg : Outport
  wires:
  bingo_dec16_32k_clr_bc_user_data_out/1 -> io_delay/1
  sim_1/1 -> convert1_1/1
  convert1_1/1 -> convert2_1/1
  convert2_1/1 -> gain_1/1
  gain_1/1 -> bingo_dec16_32k_clr_bc_user_data_out/1
  io_delay/1 -> slice_reg/1
  slice_reg/1 -> reint1/1
  reint1/1 -> in_reg/1

== system bingo_dec16_32k/cnt_rst ==
  sim_1 : Inport
  bingo_dec16_32k_cnt_rst_user_data_out : xbsIndex_r4/Gateway In  gui_display_data_type=Fixed-point  arith_type=Unsigned  n_bits=32  bin_pt=0  preci_type=Single  exp_width=8  frac_width=24  rows=1  columns=1  quantization="Round  (unbiased: +/- Inf)"  overflow=Saturate  period=1  UseAsADC=off  ADCChannel='1'  interface=None  automatic_assignment=on  address_offset=hex2dec('00')  intf_name=''  intf_description=''  default_value=0  timing_constraint=None  locs_specified=off  LOCs={}  io_standard={}  inherit_from_input=off  hdl_port=on  dbl_ovrd=off  block_type=gatewayin
  convert1_1 : DataTypeConversion  OutDataTypeStr=fixdt('ufix32_En0')  LockScale=on
  convert2_1 : DataTypeConversion  OutDataTypeStr=fixdt('ufix32_En0')  ConvertRealWorld=Stored Integer (SI)  LockScale=on
  gain_1 : Gain
  io_delay : xbsIndex_r4/Delay  rst=off  infoeditControl=Selection of Reset will increase slice count due to use of real FFs and instead of SRLs  en=off  latency=0  reg_retiming=on  dbl_ovrd=off  block_type=delay
  reint1 : xbsIndex_r4/Reinterpret  force_arith_type=on  arith_type=Unsigned  force_bin_pt=on  bin_pt=0  block_type=reinterpret
  slice_reg : xbsIndex_r4/Slice  nbits=32  boolean_output=off  mode=Lower Bit Location + Width  bit1=0  base1=MSB of Input  bit0=0  base0=LSB of Input  dbl_ovrd=off  block_type=slice
  in_reg : Outport
  wires:
  bingo_dec16_32k_cnt_rst_user_data_out/1 -> io_delay/1
  sim_1/1 -> convert1_1/1
  convert1_1/1 -> convert2_1/1
  convert2_1/1 -> gain_1/1
  gain_1/1 -> bingo_dec16_32k_cnt_rst_user_data_out/1
  io_delay/1 -> slice_reg/1
  slice_reg/1 -> reint1/1
  reint1/1 -> in_reg/1

== system bingo_dec16_32k/dest_ip ==
  sim_1 : Inport
  bingo_dec16_32k_dest_ip_user_data_out : xbsIndex_r4/Gateway In  gui_display_data_type=Fixed-point  arith_type=Unsigned  n_bits=32  bin_pt=0  preci_type=Single  exp_width=8  frac_width=24  rows=1  columns=1  quantization="Round  (unbiased: +/- Inf)"  overflow=Saturate  period=1  UseAsADC=off  ADCChannel='1'  interface=None  automatic_assignment=on  address_offset=hex2dec('00')  intf_name=''  intf_description=''  default_value=0  timing_constraint=None  locs_specified=off  LOCs={}  io_standard={}  inherit_from_input=off  hdl_port=on  dbl_ovrd=off  block_type=gatewayin
  convert1_1 : DataTypeConversion  OutDataTypeStr=fixdt('ufix32_En0')  LockScale=on
  convert2_1 : DataTypeConversion  OutDataTypeStr=fixdt('ufix32_En0')  ConvertRealWorld=Stored Integer (SI)  LockScale=on
  gain_1 : Gain
  io_delay : xbsIndex_r4/Delay  rst=off  infoeditControl=Selection of Reset will increase slice count due to use of real FFs and instead of SRLs  en=off  latency=0  reg_retiming=on  dbl_ovrd=off  block_type=delay
  reint1 : xbsIndex_r4/Reinterpret  force_arith_type=on  arith_type=Unsigned  force_bin_pt=on  bin_pt=0  block_type=reinterpret
  slice_reg : xbsIndex_r4/Slice  nbits=32  boolean_output=off  mode=Lower Bit Location + Width  bit1=0  base1=MSB of Input  bit0=0  base0=LSB of Input  dbl_ovrd=off  block_type=slice
  in_reg : Outport
  wires:
  bingo_dec16_32k_dest_ip_user_data_out/1 -> io_delay/1
  sim_1/1 -> convert1_1/1
  convert1_1/1 -> convert2_1/1
  convert2_1/1 -> gain_1/1
  gain_1/1 -> bingo_dec16_32k_dest_ip_user_data_out/1
  io_delay/1 -> slice_reg/1
  slice_reg/1 -> reint1/1
  reint1/1 -> in_reg/1

== system bingo_dec16_32k/dest_port ==
  bingo_dec16_32k_dest_port_user_data_out : xbsIndex_r4/Gateway In  gui_display_data_type=Fixed-point  arith_type=Unsigned  n_bits=32  bin_pt=0  preci_type=Single  exp_width=8  frac_width=24  rows=1  columns=1  quantization="Round  (unbiased: +/- Inf)"  overflow=Saturate  period=1  UseAsADC=off  ADCChannel='1'  interface=None  automatic_assignment=on  address_offset=hex2dec('00')  intf_name=''  intf_description=''  default_value=0  timing_constraint=None  locs_specified=off  LOCs={}  io_standard={}  inherit_from_input=off  hdl_port=on  dbl_ovrd=off  block_type=gatewayin
  convert1_1 : DataTypeConversion  OutDataTypeStr=fixdt('ufix16_En0')  LockScale=on
  convert2_1 : DataTypeConversion  OutDataTypeStr=fixdt('ufix16_En0')  ConvertRealWorld=Stored Integer (SI)  LockScale=on
  gain_1 : Gain
  io_delay : xbsIndex_r4/Delay  rst=off  infoeditControl=Selection of Reset will increase slice count due to use of real FFs and instead of SRLs  en=off  latency=0  reg_retiming=on  dbl_ovrd=off  block_type=delay
  reint1 : xbsIndex_r4/Reinterpret  force_arith_type=on  arith_type=Unsigned  force_bin_pt=on  bin_pt=0  block_type=reinterpret
  sim_1 : Constant  Value=0
  slice_reg : xbsIndex_r4/Slice  nbits=16  boolean_output=off  mode=Lower Bit Location + Width  bit1=0  base1=MSB of Input  bit0=0  base0=LSB of Input  dbl_ovrd=off  block_type=slice
  in_reg : Outport
  wires:
  bingo_dec16_32k_dest_port_user_data_out/1 -> io_delay/1
  sim_1/1 -> convert1_1/1
  convert1_1/1 -> convert2_1/1
  convert2_1/1 -> gain_1/1
  gain_1/1 -> bingo_dec16_32k_dest_port_user_data_out/1
  io_delay/1 -> slice_reg/1
  slice_reg/1 -> reint1/1
  reint1/1 -> in_reg/1

== system bingo_dec16_32k/duration ==
  sim_1 : Inport
  bingo_dec16_32k_duration_user_data_out : xbsIndex_r4/Gateway In  gui_display_data_type=Fixed-point  arith_type=Unsigned  n_bits=32  bin_pt=0  preci_type=Single  exp_width=8  frac_width=24  rows=1  columns=1  quantization="Round  (unbiased: +/- Inf)"  overflow=Saturate  period=1  UseAsADC=off  ADCChannel='1'  interface=None  automatic_assignment=on  address_offset=hex2dec('00')  intf_name=''  intf_description=''  default_value=0  timing_constraint=None  locs_specified=off  LOCs={}  io_standard={}  inherit_from_input=off  hdl_port=on  dbl_ovrd=off  block_type=gatewayin
  convert1_1 : DataTypeConversion  OutDataTypeStr=fixdt('ufix32_En0')  LockScale=on
  convert2_1 : DataTypeConversion  OutDataTypeStr=fixdt('ufix32_En0')  ConvertRealWorld=Stored Integer (SI)  LockScale=on
  gain_1 : Gain
  io_delay : xbsIndex_r4/Delay  rst=off  infoeditControl=Selection of Reset will increase slice count due to use of real FFs and instead of SRLs  en=off  latency=0  reg_retiming=on  dbl_ovrd=off  block_type=delay
  reint1 : xbsIndex_r4/Reinterpret  force_arith_type=on  arith_type=Unsigned  force_bin_pt=on  bin_pt=0  block_type=reinterpret
  slice_reg : xbsIndex_r4/Slice  nbits=32  boolean_output=off  mode=Lower Bit Location + Width  bit1=0  base1=MSB of Input  bit0=0  base0=LSB of Input  dbl_ovrd=off  block_type=slice
  in_reg : Outport
  wires:
  bingo_dec16_32k_duration_user_data_out/1 -> io_delay/1
  sim_1/1 -> convert1_1/1
  convert1_1/1 -> convert2_1/1
  convert2_1/1 -> gain_1/1
  gain_1/1 -> bingo_dec16_32k_duration_user_data_out/1
  io_delay/1 -> slice_reg/1
  slice_reg/1 -> reint1/1
  reint1/1 -> in_reg/1

== system bingo_dec16_32k/duty_cycle ==
  sim_1 : Inport
  bingo_dec16_32k_duty_cycle_user_data_out : xbsIndex_r4/Gateway In  gui_display_data_type=Fixed-point  arith_type=Unsigned  n_bits=32  bin_pt=0  preci_type=Single  exp_width=8  frac_width=24  rows=1  columns=1  quantization="Round  (unbiased: +/- Inf)"  overflow=Saturate  period=1  UseAsADC=off  ADCChannel='1'  interface=None  automatic_assignment=on  address_offset=hex2dec('00')  intf_name=''  intf_description=''  default_value=0  timing_constraint=None  locs_specified=off  LOCs={}  io_standard={}  inherit_from_input=off  hdl_port=on  dbl_ovrd=off  block_type=gatewayin
  convert1_1 : DataTypeConversion  OutDataTypeStr=fixdt('ufix32_En0')  LockScale=on
  convert2_1 : DataTypeConversion  OutDataTypeStr=fixdt('ufix32_En0')  ConvertRealWorld=Stored Integer (SI)  LockScale=on
  gain_1 : Gain
  io_delay : xbsIndex_r4/Delay  rst=off  infoeditControl=Selection of Reset will increase slice count due to use of real FFs and instead of SRLs  en=off  latency=0  reg_retiming=on  dbl_ovrd=off  block_type=delay
  reint1 : xbsIndex_r4/Reinterpret  force_arith_type=on  arith_type=Unsigned  force_bin_pt=on  bin_pt=0  block_type=reinterpret
  slice_reg : xbsIndex_r4/Slice  nbits=32  boolean_output=off  mode=Lower Bit Location + Width  bit1=0  base1=MSB of Input  bit0=0  base0=LSB of Input  dbl_ovrd=off  block_type=slice
  in_reg : Outport
  wires:
  bingo_dec16_32k_duty_cycle_user_data_out/1 -> io_delay/1
  sim_1/1 -> convert1_1/1
  convert1_1/1 -> convert2_1/1
  convert2_1/1 -> gain_1/1
  gain_1/1 -> bingo_dec16_32k_duty_cycle_user_data_out/1
  io_delay/1 -> slice_reg/1
  slice_reg/1 -> reint1/1
  reint1/1 -> in_reg/1

== system bingo_dec16_32k/dv_adc_count ==
  out_reg : Inport
  assert_reg : xbsIndex_r4/Assert  assert_type=on  type_source=Explicitly  gui_display_data_type=Fixed-point  arith_type=Unsigned  n_bits=32  bin_pt=0  preci_type=Single  exp_width=8  frac_width=24  assert_rate=off  rate_source=Explicitly  period=1  output_port=on  block_type=assert
  bingo_dec16_32k_dv_adc_count_user_data_in : xbsIndex_r4/Gateway Out  inherit_from_input=off  hdl_port=on  rows=1  columns=1  UseAsDAC=off  DACChannel='1'  interface=None  automatic_assignment=on  address_offset=hex2dec('00')  intf_name=''  intf_description=''  timing_constraint=None  locs_specified=off  LOCs={}  io_standard={}  block_type=gatewayout
  cast_gw : xbsIndex_r4/Convert  gui_display_data_type=Fixed-point  arith_type=Unsigned  n_bits=32  bin_pt=0  float_type=Single  exp_bits=8  fraction_bits=24  quantization=Truncate  overflow=Wrap  en=off  latency=1  pipeline=off  dbl_ovrd=off  block_type=convert
  io_delay : xbsIndex_r4/Delay  rst=off  infoeditControl=Selection of Reset will increase slice count due to use of real FFs and instead of SRLs  en=off  latency=0  reg_retiming=on  dbl_ovrd=off  block_type=delay
  reint1 : xbsIndex_r4/Reinterpret  force_arith_type=on  arith_type=Unsigned  force_bin_pt=on  bin_pt=0  block_type=reinterpret
  sim_out : Terminator
  sim_out_reg_gw : xbsIndex_r4/Gateway Out  inherit_from_input=off  hdl_port=off  rows=1  columns=1  UseAsDAC=off  DACChannel='1'  interface=None  automatic_assignment=on  address_offset=hex2dec('00')  intf_name=''  intf_description=''  timing_constraint=None  locs_specified=off  LOCs={}  io_standard={}  block_type=gatewayout
  sim_out_reg_sim_delay : xbsIndex_r4/Delay  rst=off  infoeditControl=Selection of Reset will increase slice count due to use of real FFs and instead of SRLs  en=off  latency=1  reg_retiming=on  dbl_ovrd=off  block_type=delay
  sim_out_reg : Outport
  wires:
  sim_out_reg_sim_delay/1 -> sim_out_reg_gw/1
  sim_out_reg_gw/1 -> sim_out_reg/1
  io_delay/1 -> cast_gw/1
  cast_gw/1 -> bingo_dec16_32k_dv_adc_count_user_data_in/1
  bingo_dec16_32k_dv_adc_count_user_data_in/1 -> sim_out/1
  out_reg/1 -> sim_out_reg_sim_delay/1, assert_reg/1
  assert_reg/1 -> reint1/1
  reint1/1 -> io_delay/1

== system bingo_dec16_32k/dv_fft_count ==
  out_reg : Inport
  assert_reg : xbsIndex_r4/Assert  assert_type=on  type_source=Explicitly  gui_display_data_type=Fixed-point  arith_type=Unsigned  n_bits=32  bin_pt=0  preci_type=Single  exp_width=8  frac_width=24  assert_rate=off  rate_source=Explicitly  period=1  output_port=on  block_type=assert
  bingo_dec16_32k_dv_fft_count_user_data_in : xbsIndex_r4/Gateway Out  inherit_from_input=off  hdl_port=on  rows=1  columns=1  UseAsDAC=off  DACChannel='1'  interface=None  automatic_assignment=on  address_offset=hex2dec('00')  intf_name=''  intf_description=''  timing_constraint=None  locs_specified=off  LOCs={}  io_standard={}  block_type=gatewayout
  cast_gw : xbsIndex_r4/Convert  gui_display_data_type=Fixed-point  arith_type=Unsigned  n_bits=32  bin_pt=0  float_type=Single  exp_bits=8  fraction_bits=24  quantization=Truncate  overflow=Wrap  en=off  latency=1  pipeline=off  dbl_ovrd=off  block_type=convert
  io_delay : xbsIndex_r4/Delay  rst=off  infoeditControl=Selection of Reset will increase slice count due to use of real FFs and instead of SRLs  en=off  latency=0  reg_retiming=on  dbl_ovrd=off  block_type=delay
  reint1 : xbsIndex_r4/Reinterpret  force_arith_type=on  arith_type=Unsigned  force_bin_pt=on  bin_pt=0  block_type=reinterpret
  sim_out : Terminator
  sim_out_reg_gw : xbsIndex_r4/Gateway Out  inherit_from_input=off  hdl_port=off  rows=1  columns=1  UseAsDAC=off  DACChannel='1'  interface=None  automatic_assignment=on  address_offset=hex2dec('00')  intf_name=''  intf_description=''  timing_constraint=None  locs_specified=off  LOCs={}  io_standard={}  block_type=gatewayout
  sim_out_reg_sim_delay : xbsIndex_r4/Delay  rst=off  infoeditControl=Selection of Reset will increase slice count due to use of real FFs and instead of SRLs  en=off  latency=1  reg_retiming=on  dbl_ovrd=off  block_type=delay
  sim_out_reg : Outport
  wires:
  sim_out_reg_sim_delay/1 -> sim_out_reg_gw/1
  sim_out_reg_gw/1 -> sim_out_reg/1
  io_delay/1 -> cast_gw/1
  cast_gw/1 -> bingo_dec16_32k_dv_fft_count_user_data_in/1
  bingo_dec16_32k_dv_fft_count_user_data_in/1 -> sim_out/1
  out_reg/1 -> sim_out_reg_sim_delay/1, assert_reg/1
  assert_reg/1 -> reint1/1
  reint1/1 -> io_delay/1

== system bingo_dec16_32k/dvout_fft_count ==
  out_reg : Inport
  assert_reg : xbsIndex_r4/Assert  assert_type=on  type_source=Explicitly  gui_display_data_type=Fixed-point  arith_type=Unsigned  n_bits=32  bin_pt=0  preci_type=Single  exp_width=8  frac_width=24  assert_rate=off  rate_source=Explicitly  period=1  output_port=on  block_type=assert
  bingo_dec16_32k_dvout_fft_count_user_data_in : xbsIndex_r4/Gateway Out  inherit_from_input=off  hdl_port=on  rows=1  columns=1  UseAsDAC=off  DACChannel='1'  interface=None  automatic_assignment=on  address_offset=hex2dec('00')  intf_name=''  intf_description=''  timing_constraint=None  locs_specified=off  LOCs={}  io_standard={}  block_type=gatewayout
  cast_gw : xbsIndex_r4/Convert  gui_display_data_type=Fixed-point  arith_type=Unsigned  n_bits=32  bin_pt=0  float_type=Single  exp_bits=8  fraction_bits=24  quantization=Truncate  overflow=Wrap  en=off  latency=1  pipeline=off  dbl_ovrd=off  block_type=convert
  io_delay : xbsIndex_r4/Delay  rst=off  infoeditControl=Selection of Reset will increase slice count due to use of real FFs and instead of SRLs  en=off  latency=0  reg_retiming=on  dbl_ovrd=off  block_type=delay
  reint1 : xbsIndex_r4/Reinterpret  force_arith_type=on  arith_type=Unsigned  force_bin_pt=on  bin_pt=0  block_type=reinterpret
  sim_out : Terminator
  sim_out_reg_gw : xbsIndex_r4/Gateway Out  inherit_from_input=off  hdl_port=off  rows=1  columns=1  UseAsDAC=off  DACChannel='1'  interface=None  automatic_assignment=on  address_offset=hex2dec('00')  intf_name=''  intf_description=''  timing_constraint=None  locs_specified=off  LOCs={}  io_standard={}  block_type=gatewayout
  sim_out_reg_sim_delay : xbsIndex_r4/Delay  rst=off  infoeditControl=Selection of Reset will increase slice count due to use of real FFs and instead of SRLs  en=off  latency=1  reg_retiming=on  dbl_ovrd=off  block_type=delay
  sim_out_reg : Outport
  wires:
  sim_out_reg_sim_delay/1 -> sim_out_reg_gw/1
  sim_out_reg_gw/1 -> sim_out_reg/1
  io_delay/1 -> cast_gw/1
  cast_gw/1 -> bingo_dec16_32k_dvout_fft_count_user_data_in/1
  bingo_dec16_32k_dvout_fft_count_user_data_in/1 -> sim_out/1
  out_reg/1 -> sim_out_reg_sim_delay/1, assert_reg/1
  assert_reg/1 -> reint1/1
  reint1/1 -> io_delay/1

== system bingo_dec16_32k/fft_shift ==
  sim_1 : Inport
  bingo_dec16_32k_fft_shift_user_data_out : xbsIndex_r4/Gateway In  gui_display_data_type=Fixed-point  arith_type=Unsigned  n_bits=32  bin_pt=0  preci_type=Single  exp_width=8  frac_width=24  rows=1  columns=1  quantization="Round  (unbiased: +/- Inf)"  overflow=Saturate  period=1  UseAsADC=off  ADCChannel='1'  interface=None  automatic_assignment=on  address_offset=hex2dec('00')  intf_name=''  intf_description=''  default_value=0  timing_constraint=None  locs_specified=off  LOCs={}  io_standard={}  inherit_from_input=off  hdl_port=on  dbl_ovrd=off  block_type=gatewayin
  convert1_1 : DataTypeConversion  OutDataTypeStr=fixdt('ufix16_En0')  LockScale=on
  convert2_1 : DataTypeConversion  OutDataTypeStr=fixdt('ufix16_En0')  ConvertRealWorld=Stored Integer (SI)  LockScale=on
  gain_1 : Gain
  io_delay : xbsIndex_r4/Delay  rst=off  infoeditControl=Selection of Reset will increase slice count due to use of real FFs and instead of SRLs  en=off  latency=0  reg_retiming=on  dbl_ovrd=off  block_type=delay
  reint1 : xbsIndex_r4/Reinterpret  force_arith_type=on  arith_type=Unsigned  force_bin_pt=on  bin_pt=0  block_type=reinterpret
  slice_reg : xbsIndex_r4/Slice  nbits=16  boolean_output=off  mode=Lower Bit Location + Width  bit1=0  base1=MSB of Input  bit0=0  base0=LSB of Input  dbl_ovrd=off  block_type=slice
  in_reg : Outport
  wires:
  bingo_dec16_32k_fft_shift_user_data_out/1 -> io_delay/1
  sim_1/1 -> convert1_1/1
  convert1_1/1 -> convert2_1/1
  convert2_1/1 -> gain_1/1
  gain_1/1 -> bingo_dec16_32k_fft_shift_user_data_out/1
  io_delay/1 -> slice_reg/1
  slice_reg/1 -> reint1/1
  reint1/1 -> in_reg/1
